simulink model "simClient"  (R2024a)
settings: Solver=FixedStepDiscrete  StartTime=0.0  StopTime=inf  FixedStep=0.001  RelTol=1e-3  EnableMultiTasking=on
libraries: quarc_library x3
settings Model: ExtModeTrigDuration=10000  Creator=mbohra  LastModifiedBy=mbohra
settings SolverCC: AlgebraicLoopSolver=TrustRegion  PositivePriorityOrder=on
settings DataIOCC: ReturnWorkspaceOutputs=off
settings DebuggingCC: UnconnectedInputMsg=warning  UnconnectedOutputMsg=warning  UnconnectedLineMsg=warning  ArithmeticOperatorsInVariantConditions=warning
settings ModelReferenceCC: EnableRefExpFcnMdlSchedulingChecks=on
settings SFSimCC: SimUseLocalCustomCode=off  CustomCodeUndefinedFunction=UseInterfaceOnly
settings RTWCC: Description=QUARC Win64 Target Using Toolchain  SystemTargetFile=quarc_win64.tlc  TemplateMakefile=quarc_default_tmf  RTWUseLocalCustomCode=off  Toolchain=QUARC win64 | nmake (64-bit Windows)  BuildConfiguration=Faster Runs  GPUComputeCapability=3.5
settings CodeAppCC: StateflowObjectComments=on
settings STFCustomTargetCC: ConcurrentExecutionCompliant=on  SystemTargetFile=quarc_win64.tlc
settings GRTTargetCC: ParMdlRefBuildCompliant=off  CompOptLevelCompliant=off  CombineOutputUpdateFcns=off  MatFileLogging=off  CPPClassGenCompliant=off  GRTInterface=on  ExtMode=on  ExtModeMexFile=quarc_comm
settings ConfigComp: CovMetricSettings=dswe

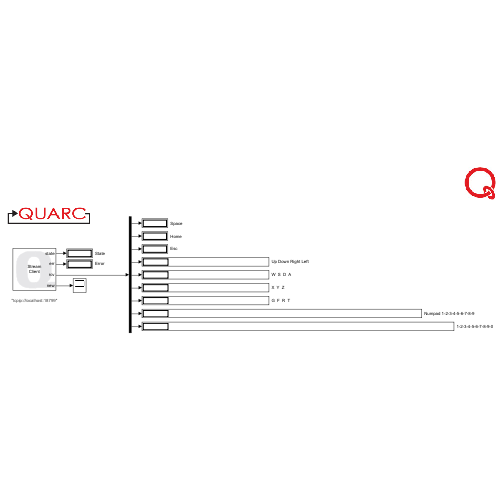
[thumbnail: Simulink's stored preview of the top-level diagram]
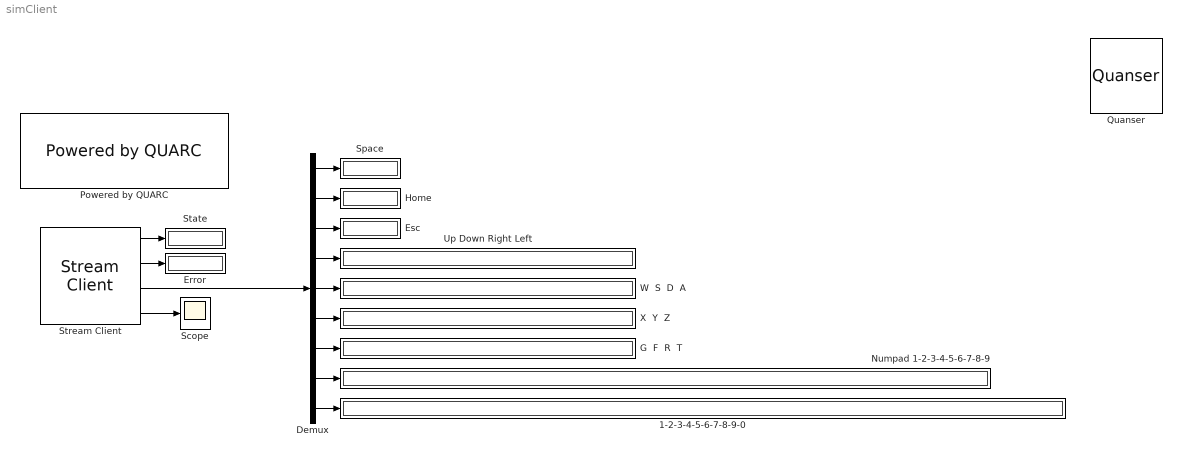
== system simClient ==
  1-2-3-4-5-6-7-8-9-0 : Display
  Demux : Demux  Outputs=[1 1 1 4 4 3 4 9 10]
  Error : Display
  Esc : Display
  G  F  R  T : Display
  Home : Display
  "Numpad 1-2-3-4-5-6-7-8-9 " : Display
  Powered by QUARC : quarc_library/Logos/Powered by QUARC
  Quanser : quarc_library/Logos/Quanser
  Scope : Scope
  Space : Display
  State : Display
  Stream Client : quarc_library/Communications/Basic/Stream Client  uri_source=Specify via dialog (do not evaluate)  uri=tcpip://localhost:18799  send_buffer_size=1460  receive_buffer_size=1460  byte_order=little endian (Intel - LSB first)  optimization=Minimum latency  send_options=Do not send data  receive_options=Receive most recent data  default_value=zeros(1,37,'logical')  sample_time=qc_get_step_size  active=off  implementation=Use non-blocking I/O  send_fifo_size=1000  receive_fifo_size=1000  send_priority=0  receive_priority=0  send_dimensions=off  receive_dimensions=off  max_dimensions=-1  data_type=boolean  type_expr=BusObject
      settings: AttributesFormatString="\"tcpip://localhost:18799\""
  Up Down Right Left : Display
  W  S  D  A : Display
  X  Y  Z : Display
  wires:
  Demux/2 -> Home/1
  Demux/3 -> Esc/1
  Demux/4 -> Up Down Right Left/1
  Demux/1 -> Space/1
  Demux/5 -> W  S  D  A/1
  Stream Client/3 -> Demux/1
  Stream Client/1 -> State/1
  Stream Client/2 -> Error/1
  Stream Client/4 -> Scope/1
  Demux/8 -> "Numpad 1-2-3-4-5-6-7-8-9 "/1
  Demux/9 -> 1-2-3-4-5-6-7-8-9-0/1
  Demux/6 -> X  Y  Z/1
  Demux/7 -> G  F  R  T/1
